simulink model "tankproblem"  (R2017b)
settings: Solver=VariableStepAuto  StartTime=0.0  StopTime=3000  RelTol=1e-3
undefined symbols (not defined in the file or in its folder): a, c, Qin
settings Model: Creator=justi  LastModifiedBy=justi

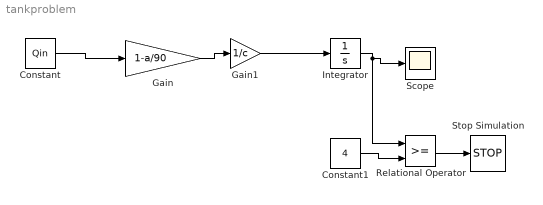
== system tankproblem ==
  Constant : Constant  Value=Qin
  Constant1 : Constant  Value=4
  Gain : Gain  Gain=1-a/90
  Gain1 : Gain  Gain=1/c
  Integrator : Integrator
  Relational Operator : RelationalOperator  OutDataTypeStr=boolean  RndMeth=Simplest
  Scope : Scope
  Stop Simulation : Stop
  wires:
  Constant/1 -> Gain/1
  Gain/1 -> Gain1/1
  Gain1/1 -> Integrator/1
  Constant1/1 -> Relational Operator/2
  Integrator/1 -> Relational Operator/1, Scope/1
  Relational Operator/1 -> Stop Simulation/1
